simulink model "two_point_dft"  (R2018a)
settings: Solver=VariableStepAuto  StartTime=0.0  StopTime=10.0  RelTol=1e-3
settings Model: Creator=eechris  LastModifiedBy=eechris

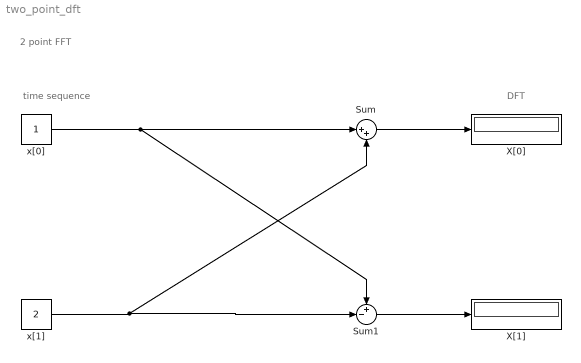
== system two_point_dft ==
  note: time sequence
  note: DFT
  note: 2 point FFT
  Sum : Sum  Inputs=|++
  Sum1 : Sum  Inputs=+-|
  X[0] : Display
  X[1] : Display
  x[0] : Constant
  x[1] : Constant  Value=2
  wires:
  Sum/1 -> X[0]/1
  Sum1/1 -> X[1]/1
  x[1]/1 -> Sum1/2, Sum/2
  x[0]/1 -> Sum1/1, Sum/1
